simulink model "TestDeriveMatlabFun2"  (R2013b)
settings: Solver=ode45  StartTime=0.0  StopTime=10.0  RelTol=1e-3
settings Model: Creator=Think79  LastModifiedBy=Think79

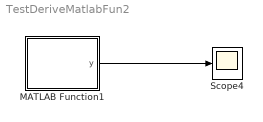
== system TestDeriveMatlabFun2 ==
  MATLAB Function1 : MATLAB Function  TreatAsAtomicUnit=on
  Scope4 : Scope
      settings: YMin=-2.25  YMax=0.75
  wires:
  MATLAB Function1/1(y) -> Scope4/1

== matlab function TestDeriveMatlabFun2/MATLAB Function1 ==
  data: y output
function y = fcn()
%#codegen
x=1:5;
y=1:5;
z=zeros(5,5);
y=interp2(x,y,z,1:5,1:5,'spline');  % worked when delete the 'spline'

end
